simulink model "intDetEx3p4p1BJDFMDL12a"  (R2015b)
settings: Solver=ode45  StartTime=0.0  StopTime=10.0  RelTol=1e-3
values from neighbouring files (symbols this model uses):
  A = -L    [intrusionDetectionMS.m]
  C = [ ... (first row only)    [intrusionDetectionMS.m]
  f1Val = 10    [intrusionDetectionMS.m]
  f2Val = 10    [intrusionDetectionMS.m]
  f3Val = 10    [intrusionDetectionMS.m]
  f4Val = 10    [intrusionDetectionMS.m]
  f5Val = 10    [intrusionDetectionMS.m]
  f6Val = 10    [intrusionDetectionMS.m]
  f7Val = 10    [intrusionDetectionMS.m]
  flt1 = 0    [intrusionDetectionMS.m]
  flt2 = 0    [intrusionDetectionMS.m]
  flt3 = 0    [intrusionDetectionMS.m]
  flt4 = 1    [intrusionDetectionMS.m]
  flt5 = 0    [intrusionDetectionMS.m]
  flt6 = 0    [intrusionDetectionMS.m]
  flt7 = 0    [intrusionDetectionMS.m]
  L = [ ... (first row only)    [intrusionDetectionMS.m]
  tf1 = 2    [intrusionDetectionMS.m]
  tf2 = 2    [intrusionDetectionMS.m]
  tf3 = 2    [intrusionDetectionMS.m]
  tf4 = 2    [intrusionDetectionMS.m]
  tf5 = 2    [intrusionDetectionMS.m]
  tf6 = 5    [intrusionDetectionMS.m]
  tf7 = 7    [intrusionDetectionMS.m]
  x0 = [0 1 1 0 0 0 0]    [intrusionDetectionMS.m]
undefined symbols (not defined in the file or in its folder): D, magnitude, pCV
settings Model: Creator=sqn4594  LastModifiedBy=samnazari
settings DataIOCC: SaveFormat=Array
settings DebuggingCC: SolverPrmCheckMsg=warning  FcnCallInpInsideContextMsg=EnableAllAsWarning
settings HardwareCC: ProdBitPerPointer=32  ProdLargestAtomicFloat=None  ProdIntDivRoundTo=Undefined  ProdEndianess=Unspecified  ProdWordSize=32  ProdHWDeviceType=32-bit Generic
settings GRTTargetCC: GeneratePreprocessorConditionals=Disable all
settings ConfigComp: CovModelRefEnable=Off

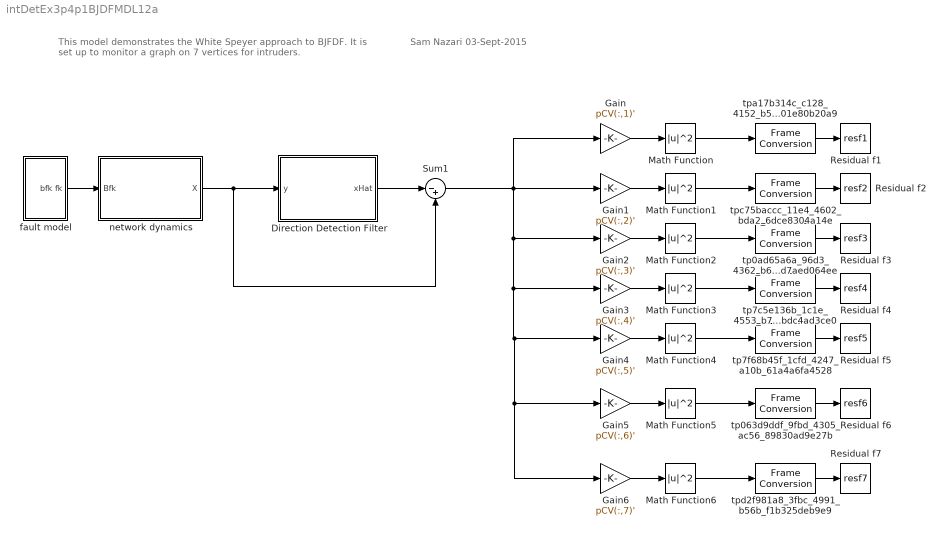
== system intDetEx3p4p1BJDFMDL12a ==
  note: Sam Nazari
      | 03-Sept-2015
  note: This model demonstrates the White Speyer approach to BJFDF.
      | It is set up to monitor a graph on 7 vertices for intruders.
  Direction Detection Filter : Subsystem
  Gain : Gain  Gain=pCV(:,1)'
  Gain1 : Gain  Gain=pCV(:,2)'
  Gain2 : Gain  Gain=pCV(:,3)'
  Gain3 : Gain  Gain=pCV(:,4)'
  Gain4 : Gain  Gain=pCV(:,5)'
  Gain5 : Gain  Gain=pCV(:,6)'
  Gain6 : Gain  Gain=pCV(:,7)'
  Math Function{,1..6} (7 alike) : Math  Operator=magnitude^2  SaturateOnIntegerOverflow=on
  Residual f1 : ToWorkspace  VariableName=resf1  SampleTime=-1
  Residual f2 : ToWorkspace  VariableName=resf2  SampleTime=-1
  Residual f3 : ToWorkspace  VariableName=resf3  SampleTime=-1
  Residual f4 : ToWorkspace  VariableName=resf4  SampleTime=-1
  Residual f5 : ToWorkspace  VariableName=resf5  SampleTime=-1
  Residual f6 : ToWorkspace  VariableName=resf6  SampleTime=-1
  Residual f7 : ToWorkspace  VariableName=resf7  SampleTime=-1
  Sum1 : Sum  Inputs=|-+
  fault model : Subsystem
  network dynamics : Subsystem
  tp063d9ddf_9fbd_4305_ac56_89830ad9e27b : FrameConversion  InheritSamplingMode=off  OutFrame=Sample-based
  tp0ad65a6a_96d3_4362_b60f_75d7aed064ee : FrameConversion  InheritSamplingMode=off  OutFrame=Sample-based
  tp7c5e136b_1c1e_4553_b73e_2dbdc4ad3ce0 : FrameConversion  InheritSamplingMode=off  OutFrame=Sample-based
  tp7f68b45f_1cfd_4247_a10b_61a4a6fa4528 : FrameConversion  InheritSamplingMode=off  OutFrame=Sample-based
  tpa17b314c_c128_4152_b5af_ab01e80b20a9 : FrameConversion  InheritSamplingMode=off  OutFrame=Sample-based
  tpc75baccc_11e4_4602_bda2_6dce8304a14e : FrameConversion  InheritSamplingMode=off  OutFrame=Sample-based
  tpd2f981a8_3fbc_4991_b56b_f1b325deb9e9 : FrameConversion  InheritSamplingMode=off  OutFrame=Sample-based
  wires:
  fault model/1(bfk fk) -> network dynamics/1(Bfk)
  network dynamics/1(X) -> Direction Detection Filter/1(y), Sum1/2
  Gain/1 -> Math Function/1
  Gain1/1 -> Math Function1/1
  Gain2/1 -> Math Function2/1
  Gain3/1 -> Math Function3/1
  Gain4/1 -> Math Function4/1
  Direction Detection Filter/1("xHat ") -> Sum1/1
  Gain5/1 -> Math Function5/1
  Gain6/1 -> Math Function6/1
  Sum1/1 -> Gain6/1, Gain5/1, Gain4/1, Gain3/1, Gain2/1, Gain/1, Gain1/1
  Math Function/1 -> tpa17b314c_c128_4152_b5af_ab01e80b20a9/1
  tpa17b314c_c128_4152_b5af_ab01e80b20a9/1 -> Residual f1/1
  Math Function1/1 -> tpc75baccc_11e4_4602_bda2_6dce8304a14e/1
  tpc75baccc_11e4_4602_bda2_6dce8304a14e/1 -> Residual f2/1
  Math Function2/1 -> tp0ad65a6a_96d3_4362_b60f_75d7aed064ee/1
  tp0ad65a6a_96d3_4362_b60f_75d7aed064ee/1 -> Residual f3/1
  Math Function3/1 -> tp7c5e136b_1c1e_4553_b73e_2dbdc4ad3ce0/1
  tp7c5e136b_1c1e_4553_b73e_2dbdc4ad3ce0/1 -> Residual f4/1
  Math Function4/1 -> tp7f68b45f_1cfd_4247_a10b_61a4a6fa4528/1
  tp7f68b45f_1cfd_4247_a10b_61a4a6fa4528/1 -> Residual f5/1
  Math Function5/1 -> tp063d9ddf_9fbd_4305_ac56_89830ad9e27b/1
  tp063d9ddf_9fbd_4305_ac56_89830ad9e27b/1 -> Residual f6/1
  Math Function6/1 -> tpd2f981a8_3fbc_4991_b56b_f1b325deb9e9/1
  tpd2f981a8_3fbc_4991_b56b_f1b325deb9e9/1 -> Residual f7/1

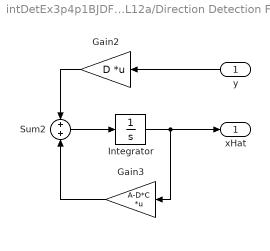
== system intDetEx3p4p1BJDFMDL12a/Direction Detection Filter ==
  y : Inport
  Gain2 : Gain  Gain=D  Multiplication=Matrix(K*u)
  Gain3 : Gain  Gain=A-D*C  Multiplication=Matrix(K*u)
  Integrator : Integrator
  Sum2 : Sum
  "xHat " : Outport
  wires:
  y/1 -> Gain2/1
  Sum2/1 -> Integrator/1
  Integrator/1 -> "xHat "/1, Gain3/1
  Gain2/1 -> Sum2/1
  Gain3/1 -> Sum2/2

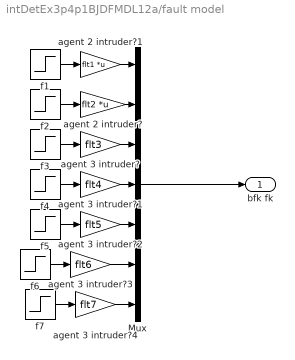
== system intDetEx3p4p1BJDFMDL12a/fault model ==
  Mux : Mux  Inputs=7
  agent 2 intruder? : Gain  Gain=flt2  Multiplication=Matrix(K*u)
  agent 2 intruder?1 : Gain  Gain=flt1  Multiplication=Matrix(K*u)
  agent 3 intruder? : Gain  Gain=flt3
  agent 3 intruder?1 : Gain  Gain=flt4
  agent 3 intruder?2 : Gain  Gain=flt5
  agent 3 intruder?3 : Gain  Gain=flt6
  agent 3 intruder?4 : Gain  Gain=flt7
  f1 : Step  After=f1Val  SampleTime=tf1
  f2 : Step  After=f2Val  SampleTime=tf2
  f3 : Step  After=f3Val  SampleTime=tf3
  f4 : Step  After=f4Val  SampleTime=tf4
  f5 : Step  After=f5Val  SampleTime=tf5
  f6 : Step  After=f6Val  SampleTime=tf6
  f7 : Step  After=f7Val  SampleTime=tf7
  bfk fk : Outport
  wires:
  Mux/1 -> bfk fk/1
  f1/1 -> agent 2 intruder?1/1
  f2/1 -> agent 2 intruder?/1
  f3/1 -> agent 3 intruder?/1
  agent 2 intruder?/1 -> Mux/2
  agent 3 intruder?/1 -> Mux/3
  agent 2 intruder?1/1 -> Mux/1
  f4/1 -> agent 3 intruder?1/1
  agent 3 intruder?1/1 -> Mux/4
  agent 3 intruder?2/1 -> Mux/5
  f5/1 -> agent 3 intruder?2/1
  f6/1 -> agent 3 intruder?3/1
  agent 3 intruder?3/1 -> Mux/6
  f7/1 -> agent 3 intruder?4/1
  agent 3 intruder?4/1 -> Mux/7

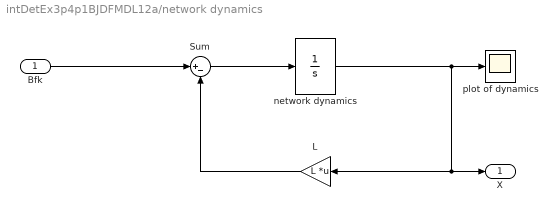
== system intDetEx3p4p1BJDFMDL12a/network dynamics ==
  Bfk : Inport
  L : Gain  Gain=L  Multiplication=Matrix(K*u)
  Sum : Sum  Inputs=|+-
  network dynamics : Integrator  InitialCondition=x0
  plot of dynamics : Scope
  X : Outport
  wires:
  Bfk/1 -> Sum/1
  Sum/1 -> network dynamics/1
  network dynamics/1 -> plot of dynamics/1, X/1, L/1
  L/1 -> Sum/2
